simulink model "v1_integral_action"  (R2023b)
settings: Solver=VariableStepAuto  StartTime=0.0  StopTime=10  RelTol=1e-3
values from neighbouring files (symbols this model uses):
  K = place(Atilde, [B; 0], [-10 -15 -20])    [WP2.m]    (also in lqr.m = lqr(sys, Qx, Qu))
settings Model: Creator=kiraa  LastModifiedBy=kiraa

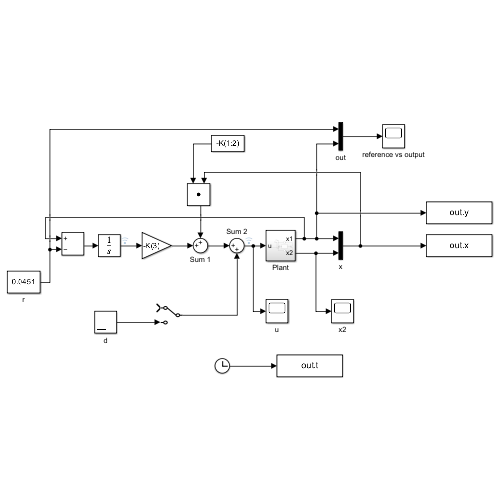
[thumbnail: Simulink's stored preview of the top-level diagram]
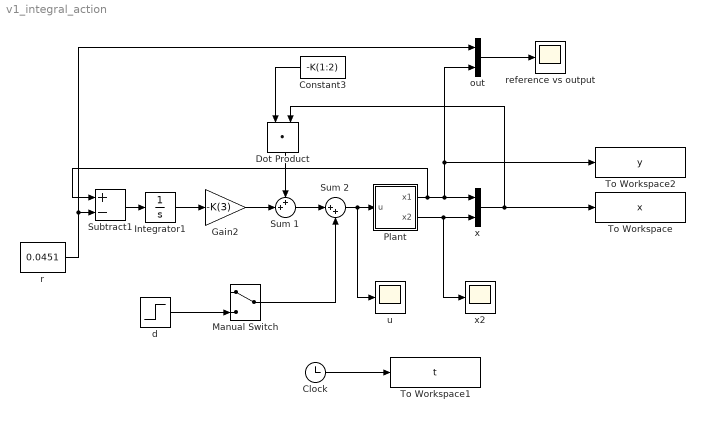
== system v1_integral_action ==
  Clock : Clock
  Constant3 : Constant  Value=-K(1:2)
  Dot Product : DotProduct  OutDataTypeStr=Inherit: Inherit via internal rule
  Gain2 : Gain  Gain=-K(3)
  Integrator1 : Integrator
  Manual Switch : ManualSwitch
  Plant : Subsystem
  Subtract1 : Sum  Inputs=+-
  Sum 1 : Sum  Inputs=++|
  Sum 2 : Sum  Inputs=|++
  To Workspace : ToWorkspace  VariableName=x  SampleTime=-1
  To Workspace1 : ToWorkspace  VariableName=t  SaveFormat=Timeseries  SampleTime=-1
  To Workspace2 : ToWorkspace  VariableName=y  SampleTime=-1
  d : Step  Time=0.5  After=20  SampleTime=0
  out : Mux  Inputs=2
  r : Constant  Value=0.0451
  reference vs output : Scope
  u : Scope
  x : Mux  Inputs=2
  x2 : Scope
  wires:
  Clock/1 -> To Workspace1/1
  Gain2/1 -> Sum 1/2
  Dot Product/1 -> Sum 1/1
  out/1 -> reference vs output/1
  Plant/1(x1) -> Subtract1/1, out/2, To Workspace2/1, x/1
  Sum 1/1 -> Sum 2/1
  Plant/2(x2) -> x2/1, x/2
  Sum 2/1 -> Plant/1(u), u/1
  d/1 -> Manual Switch/2
  Manual Switch/1 -> Sum 2/2
  Constant3/1 -> Dot Product/1
  x/1 -> To Workspace/1, Dot Product/2
  r/1 -> Subtract1/2, out/1
  Subtract1/1 -> Integrator1/1
  Integrator1/1 -> Gain2/1

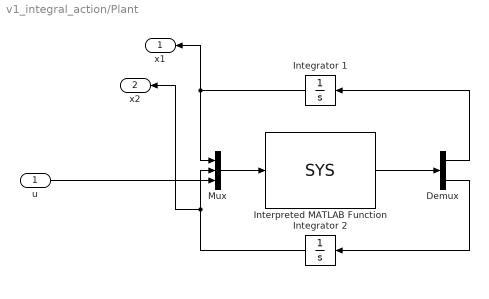
== system v1_integral_action/Plant ==
  u : Inport
  Demux : Demux  Outputs=2
  Integrator 1 : Integrator
  Integrator 2 : Integrator
  Interpreted MATLAB Function : MATLABFcn  MATLABFcn=SYS  OutputDimensions=2
  Mux : Mux  Inputs=3
  x1 : Outport
  x2 : Outport  Port=2
  wires:
  Integrator 1/1 -> x1/1, Mux/1
  Demux/1 -> Integrator 1/1
  Mux/1 -> Interpreted MATLAB Function/1
  Integrator 2/1 -> x2/1, Mux/2
  Interpreted MATLAB Function/1 -> Demux/1
  Demux/2 -> Integrator 2/1
  u/1 -> Mux/3
